simulink model "fourBar"  (Simulink 7.5)
settings: Solver=ode45  StartTime=0.0  StopTime=10.0  RelTol=1e-3
undefined symbols (not defined in the file): RootGround, RootPart
libraries: mblibv1 x13
settings Model: Creator=congyue1  LastModifiedBy=Cong Yue
settings DebuggingCC: StrictBusMsg=Warning
settings SimMechanicsCC: VisOnUpdateDiagram=on  VisDuringSimulation=on

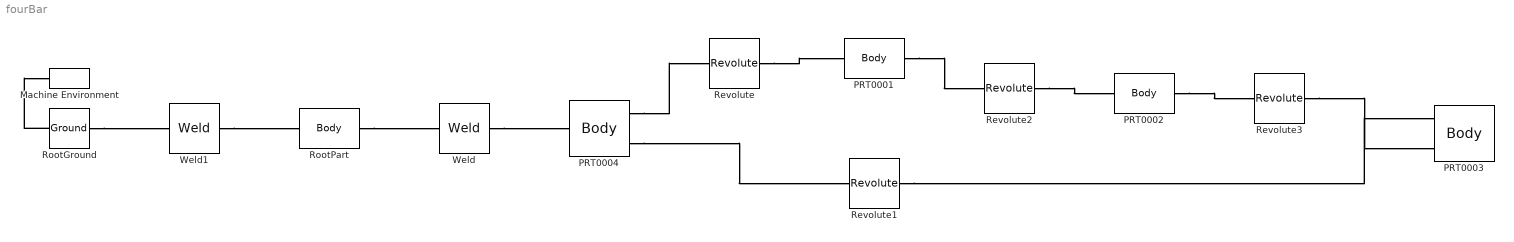
== system fourBar ==
  Machine Environment : mblibv1/Bodies/Machine Environment  DialogController=MECH.DialogSource  SystemSampleTime=-1  PortType=env  PhysicalDomain=Mechanical  DialogTemplateClass=MECH.MachineEnvironment  SyncWhenCopied=off  Gravity=[0 -9.81 0]  GravityUnits=m/s^2  GravityAsSignal=off  Dimensionality=Auto-detect  AnalysisType=Forward dynamics  LinearAssemblyTolerance=1e-3  LinearAssemblyToleranceUnits=m  AngularAssemblyTolerance=1e-3  AngularAssemblyToleranceUnits=rad  ConstraintSolverType=Stabilizing  ConstraintRelTolerance=1e-4  ConstraintAbsTolerance=1e-4  UseRobustSingularityHandling=off  RedundancyAnalysisToleranceType=Automatically select tolerance  RedundancyAnalysisTolerance=1e-14  StatePerturbationType=Fixed  PerturbationSize=1e-5  VisualizeMachine=on  BodyVisualizationType=Use model default body geometries  BodyColorSelMode=Use model default  DefaultBodyColor=[1 0 0]
  PRT0001 : mblibv1/Bodies/Body  DialogController=MECH.DynMechDlgSource  PhysicalDomain=mechanical  SubClassName=Unknown  LeftPortType=workingframe  RightPortType=workingframe  LConnTagsString=CS2  RConnTagsString=CS3  UpdateFromCAD=on  PMImportedID=40  DialogClass=MechanicalBodyBlock  Mass=1595.92  MassUnits=lbm  InertiaUnits=lbm*in^2  Inertia=[8126.51,0,-0.193068;0,386552,0;-0.193068,0,385075]  Shape=Cylinder  ShapeDims=[1 1]  ShapeUnits=m  ShapeUse=false  Density=1  DensityUnits=kg/m^3  DensityUse=false  GraphicsMode=GFXFILE  GraphicsFileName=PRT0001.stl  BodyColorSelMode=MACHINE_DEFAULT  BodyColor=[1 0 0]  AttachedToCS=CS1  CG=Right$CG$[-220.558 38.4366 7.5]$WORLD$WORLD$in$[-0.319989 0 0.947421;0.947421 0 0.319989;0 1 0]$3x3 Transform$rad$WORLD$false$40::CG(AUTOGEN)  WorkingFrames=Right$CS1$[-145.017 -110.606 5]$WORLD$WORLD$in$[-0.319989 0 0.947421;0.947421 0 0.319989;0 1 0]$3x3 Transform$rad$WORLD$false$40::CS1(AUTOGEN)#Left$CS2$[-212.558 14.7511 5]$WORLD$WORLD$in$[1 0 0;0 1 0;0 0 1]$3x3 Transform$rad$WORLD$true$39:-:40::40(AUTOGEN)#Right$CS3$[-228.557 62.1221 10]$WORLD$WORLD$in$[1 0 0;0 1 0;0 0 1]$3x3 Transform$rad$WORLD$true$40:-:41::40(AUTOGEN)  CGPos=[-220.558 38.4366 7.5]  CGRot=[-0.319989 0 0.947421;0.947421 0 0.319989;0 1 0]  CS0Pos=[]  CS0Rot=[]  CS1Pos=[-145.017 -110.606 5]  CS1Rot=[-0.319989 0 0.947421;0.947421 0 0.319989;0 1 0]  CS2Pos=[-212.558 14.7511 5]  CS2Rot=[1 0 0;0 1 0;0 0 1]  CS3Pos=[-228.557 62.1221 10]  CS3Rot=[1 0 0;0 1 0;0 0 1]  CS4Pos=[]  CS4Rot=[]  CS5Pos=[]  CS5Rot=[]  CS6Pos=[]  CS6Rot=[]  CS7Pos=[]  CS7Rot=[]  CS8Pos=[]  CS8Rot=[]  CS9Pos=[]  CS9Rot=[]  CS10Pos=[]  CS10Rot=[]  CS11Pos=[]  CS11Rot=[]  CS12Pos=[]  CS12Rot=[]  CS13Pos=[]  CS13Rot=[]  CS14Pos=[]  CS14Rot=[]  CS15Pos=[]  CS15Rot=[]  CS16Pos=[]  CS16Rot=[]  CS17Pos=[]  CS17Rot=[]  CS18Pos=[]  CS18Rot=[]  CS19Pos=[]  CS19Rot=[]  CS20Pos=[]  CS20Rot=[]
  PRT0002 : mblibv1/Bodies/Body  DialogController=MECH.DynMechDlgSource  PhysicalDomain=mechanical  SubClassName=Unknown  LeftPortType=workingframe  RightPortType=workingframe  LConnTagsString=CS2  RConnTagsString=CS3  UpdateFromCAD=on  PMImportedID=41  DialogClass=MechanicalBodyBlock  Mass=2485.02  MassUnits=lbm  InertiaUnits=lbm*in^2  Inertia=[12670,0.413616,0;0.413616,1.43591e+006,0;0,0,1.43822e+006]  Shape=Cylinder  ShapeDims=[1 1]  ShapeUnits=m  ShapeUse=false  Density=1  DensityUnits=kg/m^3  DensityUse=false  GraphicsMode=GFXFILE  GraphicsFileName=PRT0002.stl  BodyColorSelMode=MACHINE_DEFAULT  BodyColor=[1 0 0]  AttachedToCS=CS1  CG=Right$CG$[-210.88 98.0041 12.5]$WORLD$WORLD$in$[0.44193 -0.89705 0;0.89705 0.44193 0;0 0 1]$3x3 Transform$rad$WORLD$false$41::CG(AUTOGEN)  WorkingFrames=Right$CS1$[-161.836 118.433 10]$WORLD$WORLD$in$[0.44193 -0.89705 0;0.89705 0.44193 0;0 0 1]$3x3 Transform$rad$WORLD$false$41::CS1(AUTOGEN)#Left$CS2$[-228.557 62.1221 10]$WORLD$WORLD$in$[1 0 0;0 1 0;0 0 1]$3x3 Transform$rad$WORLD$true$40:-:41::41(AUTOGEN)#Right$CS3$[-193.203 133.886 10]$WORLD$WORLD$in$[1 0 0;0 1 0;0 0 1]$3x3 Transform$rad$WORLD$true$41:-:45::41(AUTOGEN)  CGPos=[-210.88 98.0041 12.5]  CGRot=[0.44193 -0.89705 0;0.89705 0.44193 0;0 0 1]  CS0Pos=[]  CS0Rot=[]  CS1Pos=[-161.836 118.433 10]  CS1Rot=[0.44193 -0.89705 0;0.89705 0.44193 0;0 0 1]  CS2Pos=[-228.557 62.1221 10]  CS2Rot=[1 0 0;0 1 0;0 0 1]  CS3Pos=[-193.203 133.886 10]  CS3Rot=[1 0 0;0 1 0;0 0 1]  CS4Pos=[]  CS4Rot=[]  CS5Pos=[]  CS5Rot=[]  CS6Pos=[]  CS6Rot=[]  CS7Pos=[]  CS7Rot=[]  CS8Pos=[]  CS8Rot=[]  CS9Pos=[]  CS9Rot=[]  CS10Pos=[]  CS10Rot=[]  CS11Pos=[]  CS11Rot=[]  CS12Pos=[]  CS12Rot=[]  CS13Pos=[]  CS13Rot=[]  CS14Pos=[]  CS14Rot=[]  CS15Pos=[]  CS15Rot=[]  CS16Pos=[]  CS16Rot=[]  CS17Pos=[]  CS17Rot=[]  CS18Pos=[]  CS18Rot=[]  CS19Pos=[]  CS19Rot=[]  CS20Pos=[]  CS20Rot=[]
  PRT0003 : mblibv1/Bodies/Body  DialogController=MECH.DynMechDlgSource  PhysicalDomain=mechanical  SubClassName=Unknown  LeftPortType=workingframe  RightPortType=workingframe  LConnTagsString=CS2|CS3  UpdateFromCAD=on  PMImportedID=45  DialogClass=MechanicalBodyBlock  Mass=6073.19  MassUnits=lbm  InertiaUnits=lbm*in^2  Inertia=[30933.7,2.09331,0;2.09331,2.07808e+007,0;0,0,2.07865e+007]  Shape=Cylinder  ShapeDims=[1 1]  ShapeUnits=m  ShapeUse=false  Density=1  DensityUnits=kg/m^3  DensityUse=false  GraphicsMode=GFXFILE  GraphicsFileName=PRT0003.stl  BodyColorSelMode=MACHINE_DEFAULT  BodyColor=[1 0 0]  AttachedToCS=CS1  CG=Right$CG$[-112.88 74.3186 7.5]$WORLD$WORLD$in$[0.803225 0.595675 0;-0.595675 0.803225 0;0 0 1]$3x3 Transform$rad$WORLD$false$45::CG(AUTOGEN)  WorkingFrames=Right$CS1$[-274.811 216.462 5]$WORLD$WORLD$in$[0.803225 0.595675 0;-0.595675 0.803225 0;0 0 1]$3x3 Transform$rad$WORLD$false$45::CS1(AUTOGEN)#Left$CS2$[-32.5579 14.7511 5]$WORLD$WORLD$in$[1 0 0;0 1 0;0 0 1]$3x3 Transform$rad$WORLD$true$39:-:45::45(AUTOGEN)#Left$CS3$[-193.203 133.886 10]$WORLD$WORLD$in$[1 0 0;0 1 0;0 0 1]$3x3 Transform$rad$WORLD$true$41:-:45::45(AUTOGEN)  CGPos=[-112.88 74.3186 7.5]  CGRot=[0.803225 0.595675 0;-0.595675 0.803225 0;0 0 1]  CS0Pos=[]  CS0Rot=[]  CS1Pos=[-274.811 216.462 5]  CS1Rot=[0.803225 0.595675 0;-0.595675 0.803225 0;0 0 1]  CS2Pos=[-32.5579 14.7511 5]  CS2Rot=[1 0 0;0 1 0;0 0 1]  CS3Pos=[-193.203 133.886 10]  CS3Rot=[1 0 0;0 1 0;0 0 1]  CS4Pos=[]  CS4Rot=[]  CS5Pos=[]  CS5Rot=[]  CS6Pos=[]  CS6Rot=[]  CS7Pos=[]  CS7Rot=[]  CS8Pos=[]  CS8Rot=[]  CS9Pos=[]  CS9Rot=[]  CS10Pos=[]  CS10Rot=[]  CS11Pos=[]  CS11Rot=[]  CS12Pos=[]  CS12Rot=[]  CS13Pos=[]  CS13Rot=[]  CS14Pos=[]  CS14Rot=[]  CS15Pos=[]  CS15Rot=[]  CS16Pos=[]  CS16Rot=[]  CS17Pos=[]  CS17Rot=[]  CS18Pos=[]  CS18Rot=[]  CS19Pos=[]  CS19Rot=[]  CS20Pos=[]  CS20Rot=[]
  PRT0004 : mblibv1/Bodies/Body  DialogController=MECH.DynMechDlgSource  PhysicalDomain=mechanical  SubClassName=Unknown  LeftPortType=workingframe  RightPortType=workingframe  LConnTagsString=CS2  RConnTagsString=CS3|CS4  UpdateFromCAD=on  PMImportedID=39  DialogClass=MechanicalBodyBlock  Mass=4527.49  MassUnits=lbm  InertiaUnits=lbm*in^2  Inertia=[18921,1.31502,0;1.31502,1.2401e+007,0;0,0,1.2401e+007]  Shape=Cylinder  ShapeDims=[1 1]  ShapeUnits=m  ShapeUse=false  Density=1  DensityUnits=kg/m^3  DensityUse=false  GraphicsMode=GFXFILE  GraphicsFileName=PRT0004.stl  BodyColorSelMode=MACHINE_DEFAULT  BodyColor=[1 0 0]  AttachedToCS=CS1  CG=Right$CG$[-122.558 14.7511 2.5]$WORLD$WORLD$in$[1 0 0;0 1 0;0 0 1]$3x3 Transform$rad$WORLD$false$39::CG(AUTOGEN)  WorkingFrames=Right$CS1$[0 0 0]$WORLD$WORLD$in$[1 0 0;0 1 0;0 0 1]$3x3 Transform$rad$WORLD$false$39::CS1(AUTOGEN)#Left$CS2$[-122.558 14.7511 2.5]$WORLD$WORLD$in$[1 0 0;0 1 0;0 0 1]$3x3 Transform$rad$WORLD$true$39:-:RootPart::39(AUTOGEN)#Right$CS3$[-212.558 14.7511 5]$WORLD$WORLD$in$[1 0 0;0 1 0;0 0 1]$3x3 Transform$rad$WORLD$true$39:-:40::39(AUTOGEN)#Right$CS4$[-32.5579 14.7511 5]$WORLD$WORLD$in$[1 0 0;0 1 0;0 0 1]$3x3 Transform$rad$WORLD$true$39:-:45::39(AUTOGEN)  CGPos=[-122.558 14.7511 2.5]  CGRot=[1 0 0;0 1 0;0 0 1]  CS0Pos=[]  CS0Rot=[]  CS1Pos=[0 0 0]  CS1Rot=[1 0 0;0 1 0;0 0 1]  CS2Pos=[-122.558 14.7511 2.5]  CS2Rot=[1 0 0;0 1 0;0 0 1]  CS3Pos=[-212.558 14.7511 5]  CS3Rot=[1 0 0;0 1 0;0 0 1]  CS4Pos=[-32.5579 14.7511 5]  CS4Rot=[1 0 0;0 1 0;0 0 1]  CS5Pos=[]  CS5Rot=[]  CS6Pos=[]  CS6Rot=[]  CS7Pos=[]  CS7Rot=[]  CS8Pos=[]  CS8Rot=[]  CS9Pos=[]  CS9Rot=[]  CS10Pos=[]  CS10Rot=[]  CS11Pos=[]  CS11Rot=[]  CS12Pos=[]  CS12Rot=[]  CS13Pos=[]  CS13Rot=[]  CS14Pos=[]  CS14Rot=[]  CS15Pos=[]  CS15Rot=[]  CS16Pos=[]  CS16Rot=[]  CS17Pos=[]  CS17Rot=[]  CS18Pos=[]  CS18Rot=[]  CS19Pos=[]  CS19Rot=[]  CS20Pos=[]  CS20Rot=[]
  Revolute : mblibv1/Joints/Revolute  DialogController=MECH.DynMechDlgSource  PhysicalDomain=mechanical  SubClassName=Unknown  LeftPortType=blob  RightPortType=blob  LConnTagsString=__newl0  RConnTagsString=__newr0  UpdateFromCAD=on  PMImportedID=39:-:40  NumSAPorts=0  CutJoint=off  MarkAsCut=off  Primitives=prismatic  PrimitiveProps=R1$WORLD$[0,0,-1]$revolute  DialogClass=JointBlock  R1Axis=[0,0,-1]
  Revolute1 : mblibv1/Joints/Revolute  DialogController=MECH.DynMechDlgSource  PhysicalDomain=mechanical  SubClassName=Unknown  LeftPortType=blob  RightPortType=blob  LConnTagsString=__newl0  RConnTagsString=__newr0  UpdateFromCAD=on  PMImportedID=39:-:45  NumSAPorts=0  CutJoint=off  MarkAsCut=off  Primitives=prismatic  PrimitiveProps=R1$WORLD$[0,0,-1]$revolute  DialogClass=JointBlock  R1Axis=[0,0,-1]
  Revolute2 : mblibv1/Joints/Revolute  DialogController=MECH.DynMechDlgSource  PhysicalDomain=mechanical  SubClassName=Unknown  LeftPortType=blob  RightPortType=blob  LConnTagsString=__newl0  RConnTagsString=__newr0  UpdateFromCAD=on  PMImportedID=40:-:41  NumSAPorts=0  CutJoint=off  MarkAsCut=off  Primitives=prismatic  PrimitiveProps=R1$WORLD$[0,0,-1]$revolute  DialogClass=JointBlock  R1Axis=[0,0,-1]
  Revolute3 : mblibv1/Joints/Revolute  DialogController=MECH.DynMechDlgSource  PhysicalDomain=mechanical  SubClassName=Unknown  LeftPortType=blob  RightPortType=blob  LConnTagsString=__newl0  RConnTagsString=__newr0  UpdateFromCAD=on  PMImportedID=41:-:45  NumSAPorts=0  CutJoint=off  MarkAsCut=off  Primitives=prismatic  PrimitiveProps=R1$WORLD$[0,0,-1]$revolute  DialogClass=JointBlock  R1Axis=[0,0,-1]
  RootGround : mblibv1/Bodies/Ground  DialogController=MECH.DynMechDlgSource  SystemSampleTime=-1  UpdateFromCAD=on  PMImportedID=RootGround  LeftPortType=env  RightPortType=workingframe  PhysicalDomain=Mechanical  DialogClass=GroundBlock  CoordPosition=[-144.157,56.0579,6.80441]  CoordPositionUnits=in  StateVectorMgrId=0  MachineId=[1 0]  ShowEnvPort=on
  RootPart : mblibv1/Bodies/Body  DialogController=MECH.DynMechDlgSource  PhysicalDomain=mechanical  SubClassName=Unknown  LeftPortType=workingframe  RightPortType=workingframe  LConnTagsString=CS3  RConnTagsString=CS2  UpdateFromCAD=on  PMImportedID=RootPart  DialogClass=MechanicalBodyBlock  Mass=0  MassUnits=lbm  InertiaUnits=lbm*in^2  Inertia=[0,0,0;0,0,0;0,0,0]  Shape=Cylinder  ShapeDims=[1 1]  ShapeUnits=m  ShapeUse=false  Density=1  DensityUnits=kg/m^3  DensityUse=false  GraphicsMode=MACHINE_DEFAULT  BodyColorSelMode=MACHINE_DEFAULT  BodyColor=[1 0 0]  AttachedToCS=CS1  CG=Right$CG$[-144.157 56.0579 6.80441]$WORLD$WORLD$in$[1 0 0;0 1 0;0 0 1]$3x3 Transform$rad$WORLD$false$RootPart::CG(AUTOGEN)  WorkingFrames=Right$CS1$[0 0 0]$WORLD$WORLD$in$[1 0 0;0 1 0;0 0 1]$3x3 Transform$rad$WORLD$false$RootPart::CS1(AUTOGEN)#Right$CS2$[-122.558 14.7511 2.5]$WORLD$WORLD$in$[1 0 0;0 1 0;0 0 1]$3x3 Transform$rad$WORLD$true$39:-:RootPart::RootPart(AUTOGEN)#Left$CS3$[-144.157 56.0579 6.80441]$WORLD$WORLD$in$[1 0 0;0 1 0;0 0 1]$3x3 Transform$rad$WORLD$true$RootGround:-:RootPart::RootPart(AUTOGEN)  CGPos=[-144.157 56.0579 6.80441]  CGRot=[1 0 0;0 1 0;0 0 1]  CS0Pos=[]  CS0Rot=[]  CS1Pos=[0 0 0]  CS1Rot=[1 0 0;0 1 0;0 0 1]  CS2Pos=[-122.558 14.7511 2.5]  CS2Rot=[1 0 0;0 1 0;0 0 1]  CS3Pos=[-144.157 56.0579 6.80441]  CS3Rot=[1 0 0;0 1 0;0 0 1]  CS4Pos=[]  CS4Rot=[]  CS5Pos=[]  CS5Rot=[]  CS6Pos=[]  CS6Rot=[]  CS7Pos=[]  CS7Rot=[]  CS8Pos=[]  CS8Rot=[]  CS9Pos=[]  CS9Rot=[]  CS10Pos=[]  CS10Rot=[]  CS11Pos=[]  CS11Rot=[]  CS12Pos=[]  CS12Rot=[]  CS13Pos=[]  CS13Rot=[]  CS14Pos=[]  CS14Rot=[]  CS15Pos=[]  CS15Rot=[]  CS16Pos=[]  CS16Rot=[]  CS17Pos=[]  CS17Rot=[]  CS18Pos=[]  CS18Rot=[]  CS19Pos=[]  CS19Rot=[]  CS20Pos=[]  CS20Rot=[]
  Weld : mblibv1/Joints/Weld  DialogController=MECH.DynMechDlgSource  PhysicalDomain=mechanical  SubClassName=Unknown  LeftPortType=blob  RightPortType=blob  LConnTagsString=__newl0  RConnTagsString=__newr0  UpdateFromCAD=on  PMImportedID=39:-:RootPart  NumSAPorts=0  CutJoint=off  MarkAsCut=off  Primitives=weld  PrimitiveProps=W$WORLD$[0.57735,0.57735,0.57735]$weld  DialogClass=JointBlock  WAxis=[0.57735,0.57735,0.57735]
  Weld1 : mblibv1/Joints/Weld  DialogController=MECH.DynMechDlgSource  PhysicalDomain=mechanical  SubClassName=Unknown  LeftPortType=blob  RightPortType=blob  LConnTagsString=__newl0  RConnTagsString=__newr0  UpdateFromCAD=on  PMImportedID=RootGround:-:RootPart  NumSAPorts=0  CutJoint=off  MarkAsCut=off  Primitives=weld  PrimitiveProps=W$WORLD$[0.57735,0.57735,0.57735]$weld  DialogClass=JointBlock  WAxis=[0.57735,0.57735,0.57735]
  connections:
  RootPart/RConn1 -- Weld/LConn1
  Weld/RConn1 -- PRT0004/LConn1
  PRT0004/RConn1 -- Revolute/LConn1
  Revolute/RConn1 -- PRT0001/LConn1
  PRT0004/RConn2 -- Revolute1/LConn1
  Revolute1/RConn1 -- PRT0003/LConn1
  PRT0001/RConn1 -- Revolute2/LConn1
  Revolute2/RConn1 -- PRT0002/LConn1
  PRT0002/RConn1 -- Revolute3/LConn1
  Revolute3/RConn1 -- PRT0003/LConn2
  RootGround/RConn1 -- Weld1/LConn1
  Weld1/RConn1 -- RootPart/LConn1
  RootGround/LConn1 -- Machine Environment/RConn1
